simulink model "StepperMotorMusicPulseOutput4"  (R2019b)
settings: Solver=FixedStepDiscrete  StartTime=0.0  StopTime=t_sim  FixedStep=T_s  RelTol=1e-3  EnableMultiTasking=on
undefined symbols (not defined in the file): T_s, t_sim
libraries: dspsigops x10, sbox2 x3
settings Model: Creator=haketa  LastModifiedBy=STEPPERMOTOR
settings DataIOCC: LimitDataPoints=on  SaveFormat=Array  SignalLoggingSaveFormat=ModelDataLogs  ReturnWorkspaceOutputs=off
settings OptimizationCC: BlockReduction=off  OptimizeBlockIOStorage=off  BufferReuse=off  GlobalBufferReuse=off  ExpressionFolding=off  ExpressionDepthLimit=2147483647  LocalBlockOutputs=off  InitFltsAndDblsToZero=on  LifeSpan=inf  OptimizeDataStoreBuffers=off  BusAssignmentInplaceUpdate=off
settings DebuggingCC: SaveWithParameterizedLinksMsg=none  UnderspecifiedInitializationDetection=Classic  MergeDetectMultiDrivingBlocksExec=none  SignalResolutionControl=TryResolveAllWithWarning  SolverPrmCheckMsg=warning  InheritedTsInSrcMsg=none  MultiTaskDSMMsg=warning  MultiTaskCondExecSysMsg=none  FcnCallInpInsideContextMsg=warning  StateNameClashWarn=warning  SFUnexpectedBacktrackingDiag=warning  SFNoUnconditionalDefaultTransitionDiag=warning  SFExecutionAtInitializationDiag=none  ArithmeticOperatorsInVariantConditions=warning
settings HardwareCC: ProdBitPerPointer=32  ProdBitPerSizeT=32  ProdBitPerPtrDiffT=32  ProdLargestAtomicFloat=None  ProdIntDivRoundTo=Undefined  ProdEndianess=Unspecified  ProdWordSize=32  ProdHWDeviceType=32-bit Generic
settings ModelReferenceCC: PropagateSignalLabelsOutOfModel=off
settings SFSimCC: SimUseLocalCustomCode=off  CustomCodeUndefinedFunction=UseInterfaceOnly
settings RTWCC: Description=MTT sBOXII Real-Time Target.  SystemTargetFile=sbox2.tlc  TemplateMakefile=sbox2.tmf  RTWUseLocalCustomCode=off  RTWCompilerOptimization=on
settings CodeAppCC: StateflowObjectComments=on
settings GRTTargetCC: TargetLangStandard=C89/C90 (ANSI)  GeneratePreprocessorConditionals=Disable all  MatFileLogging=off  UseToolchainInfoCompliant=off  RTWCAPISignals=on  RTWCAPIParams=on
settings ConfigComp: CovMetricSettings=dw  CovHtmlReporting=on  CovSaveCumulativeToWorkspaceVar=on  CovSaveSingleToWorkspaceVar=on  CovExternalEMLEnable=off  CovSFcnEnable=off

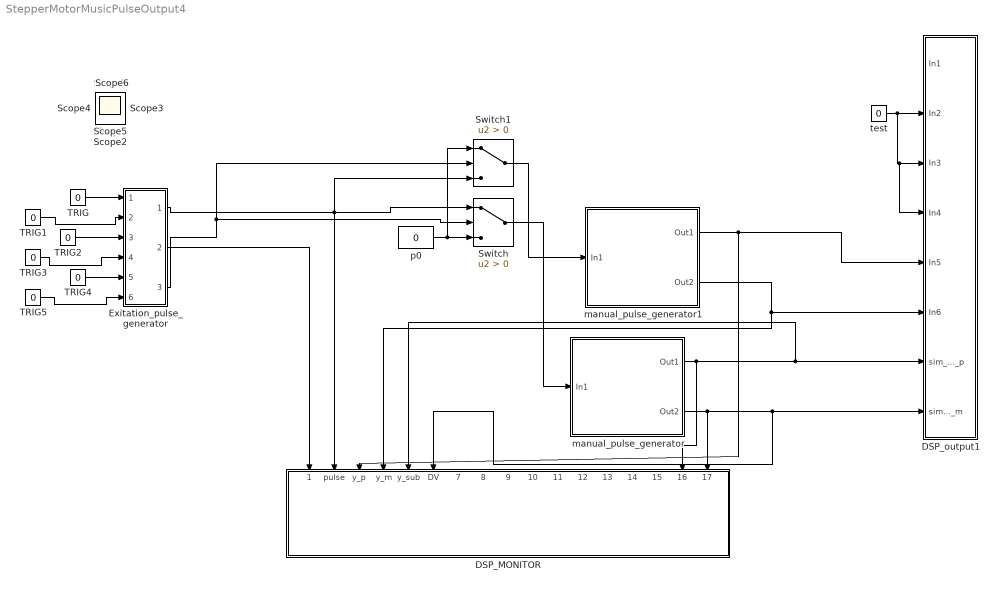
== system StepperMotorMusicPulseOutput4 ==
  DSP_MONITOR : Subsystem
  DSP_output1 : Subsystem
  Exitation_pulse_generator : Subsystem
  Switch : Switch  Criteria=u2 > Threshold
  Switch1 : Switch  Criteria=u2 > Threshold
  TRIG{,1..5} (6 alike) : Constant  Value=0  SampleTime=-1
  manual_pulse_generator : Subsystem
  manual_pulse_generator1 : Subsystem
  p0 : Constant  Value=0  SampleTime=-1
  test : Constant  Value=0  SampleTime=-1
  Scope{,1..6} (7 alike) : Scope
  wires:
  TRIG/1 -> Exitation_pulse_generator/1(TRIG)
  TRIG1/1 -> Exitation_pulse_generator/2(In2)
  TRIG3/1 -> Exitation_pulse_generator/4(In4)
  manual_pulse_generator/2(Out2) -> DSP_MONITOR/6(DV), DSP_output1/8(sim_CW_m), DSP_MONITOR/17(hoge2)
  manual_pulse_generator/1(Out1) -> DSP_output1/7(sim_CW_p), DSP_MONITOR/5(y_sub), DSP_MONITOR/16(hoge1)
  Exitation_pulse_generator/2(TRIG_parameter) -> DSP_MONITOR/1(DSP_SAVE_TRIG)
  Exitation_pulse_generator/1(sim_CW) -> Switch/1, Switch1/3, DSP_MONITOR/2(pulse)
  test/1 -> DSP_output1/2(In2), DSP_output1/3(In3), DSP_output1/4(In4)
  TRIG2/1 -> Exitation_pulse_generator/3(In3)
  TRIG4/1 -> Exitation_pulse_generator/5(In5)
  TRIG5/1 -> Exitation_pulse_generator/6(CW_p)
  Exitation_pulse_generator/3("Rot ") -> Switch/2, Switch1/2
  p0/1 -> Switch1/1, Switch/3
  Switch1/1 -> manual_pulse_generator1/1(In1)
  Switch/1 -> manual_pulse_generator/1(In1)
  manual_pulse_generator1/1(Out1) -> DSP_output1/5(In5), DSP_MONITOR/3(y_p)
  manual_pulse_generator1/2(Out2) -> DSP_MONITOR/4(y_m), DSP_output1/6(In6)

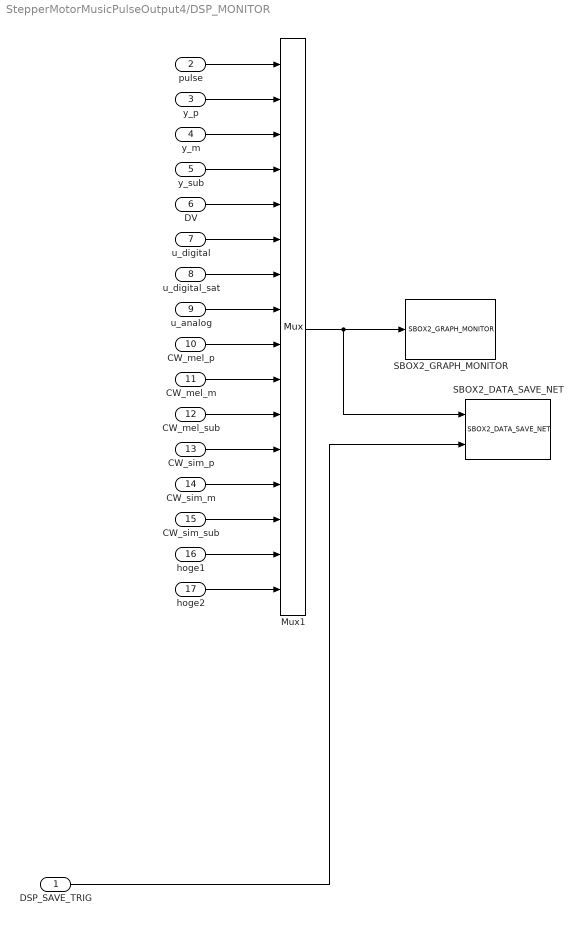
== system StepperMotorMusicPulseOutput4/DSP_MONITOR ==
  DSP_SAVE_TRIG : Inport
  pulse : Inport  Port=2
  y_p : Inport  Port=3
  y_m : Inport  Port=4
  y_sub : Inport  Port=5
  DV : Inport  Port=6
  u_digital : Inport  Port=7
  u_digital_sat : Inport  Port=8
  u_analog : Inport  Port=9
  CW_mel_p : Inport  Port=10
  CW_mel_m : Inport  Port=11
  CW_mel_sub : Inport  Port=12
  CW_sim_p : Inport  Port=13
  CW_sim_m : Inport  Port=14
  CW_sim_sub : Inport  Port=15
  hoge1 : Inport  Port=16
  hoge2 : Inport  Port=17
  Mux1 : Mux  Inputs=16
  SBOX2_DATA_SAVE_NET : sbox2/Network Data Save Devices/SBOX2_DATA_SAVE_NET  save_mode=ホストアプリケーション指示によるトリガ待ち  data_length=(t_sim/T_s)  pre_triger=0  sampletime=-1
  SBOX2_GRAPH_MONITOR : sbox2/Network Data Save Devices/SBOX2_GRAPH_MONITOR  sampletime=-1
  wires:
  DSP_SAVE_TRIG/1 -> SBOX2_DATA_SAVE_NET/2
  y_p/1 -> Mux1/2
  Mux1/1 -> SBOX2_DATA_SAVE_NET/1, SBOX2_GRAPH_MONITOR/1
  pulse/1 -> Mux1/1
  y_sub/1 -> Mux1/4
  u_digital/1 -> Mux1/6
  u_analog/1 -> Mux1/8
  u_digital_sat/1 -> Mux1/7
  DV/1 -> Mux1/5
  y_m/1 -> Mux1/3
  CW_mel_p/1 -> Mux1/9
  CW_mel_m/1 -> Mux1/10
  CW_mel_sub/1 -> Mux1/11
  CW_sim_p/1 -> Mux1/12
  CW_sim_m/1 -> Mux1/13
  CW_sim_sub/1 -> Mux1/14
  hoge1/1 -> Mux1/15
  hoge2/1 -> Mux1/16

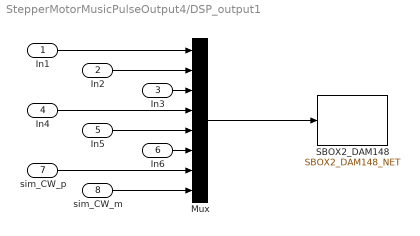
== system StepperMotorMusicPulseOutput4/DSP_output1 ==
  In1 : Inport
  In2 : Inport  Port=2
  In3 : Inport  Port=3
  In4 : Inport  Port=4
  In5 : Inport  Port=5
  In6 : Inport  Port=6
  sim_CW_p : Inport  Port=7
  sim_CW_m : Inport  Port=8
  Mux : Mux  Inputs=8
  SBOX2_DAM148 : sbox2/Analog I//O Devices/SBOX2_DAM148_NET  daStopCtrl1=0V出力  daStopCtrl2=0V出力  daStopCtrl3=0V出力  daStopCtrl4=0V出力  daStopCtrl5=0V出力  daStopCtrl6=0V出力  daStopCtrl7=0V出力  daStopCtrl8=0V出力  sampletime=-1
  wires:
  sim_CW_p/1 -> Mux/7
  Mux/1 -> SBOX2_DAM148/1
  In2/1 -> Mux/2
  In1/1 -> Mux/1
  In4/1 -> Mux/4
  In5/1 -> Mux/5
  In6/1 -> Mux/6
  sim_CW_m/1 -> Mux/8
  In3/1 -> Mux/3

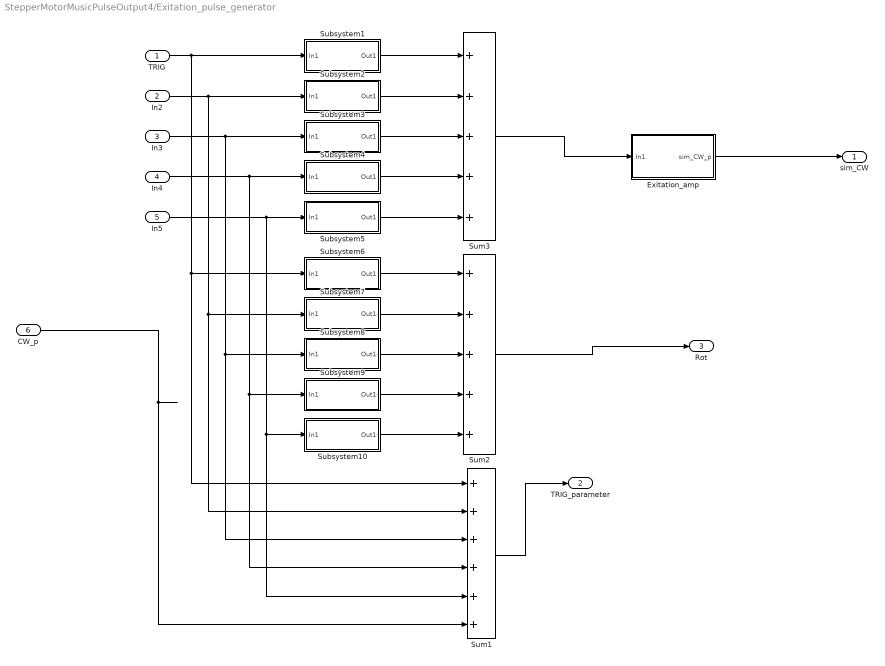
== system StepperMotorMusicPulseOutput4/Exitation_pulse_generator ==
  TRIG : Inport
  In2 : Inport  Port=2
  In3 : Inport  Port=3
  In4 : Inport  Port=4
  In5 : Inport  Port=5
  CW_p : Inport  Port=6
  Exitation_amp : Subsystem
  Subsystem1 : Subsystem
  Subsystem10 : Subsystem
  Subsystem2 : Subsystem
  Subsystem3 : Subsystem
  Subsystem4 : Subsystem
  Subsystem5 : Subsystem
  Subsystem6 : Subsystem
  Subsystem7 : Subsystem
  Subsystem8 : Subsystem
  Subsystem9 : Subsystem
  Sum1 : Sum  Inputs=++++++
  Sum2 : Sum  Inputs=+++++
  Sum3 : Sum  Inputs=+++++
  sim_CW : Outport
  TRIG_parameter : Outport  Port=2
  "Rot " : Outport  Port=3
  wires:
  Sum3/1 -> Exitation_amp/1(In1)
  Exitation_amp/1(sim_CW_p) -> sim_CW/1
  Subsystem1/1(Out1) -> Sum3/1
  In2/1 -> Subsystem2/1(In1), Sum1/2, Subsystem7/1(In1)
  In3/1 -> Subsystem3/1(In1), Subsystem8/1(In1), Sum1/3
  In4/1 -> Subsystem4/1(In1), Sum1/4, Subsystem9/1(In1)
  In5/1 -> Subsystem5/1(In1), Subsystem10/1(In1), Sum1/5
  CW_p/1 -> Sum1/6
  Subsystem2/1(Out1) -> Sum3/2
  Subsystem3/1(Out1) -> Sum3/3
  Subsystem4/1(Out1) -> Sum3/4
  Subsystem5/1(Out1) -> Sum3/5
  TRIG/1 -> Subsystem1/1(In1), Sum1/1, Subsystem6/1(In1)
  Subsystem7/1(Out1) -> Sum2/2
  Subsystem8/1(Out1) -> Sum2/3
  Subsystem9/1(Out1) -> Sum2/4
  Sum1/1 -> TRIG_parameter/1
  Subsystem10/1(Out1) -> Sum2/5
  Subsystem6/1(Out1) -> Sum2/1
  Sum2/1 -> "Rot "/1

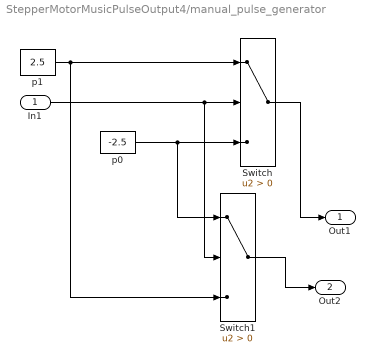
== system StepperMotorMusicPulseOutput4/manual_pulse_generator ==
  In1 : Inport
  Switch : Switch  Criteria=u2 > Threshold
  Switch1 : Switch  Criteria=u2 > Threshold
  p0 : Constant  Value=-2.5  SampleTime=-1
  p1 : Constant  Value=2.5  SampleTime=-1
  Out1 : Outport
  Out2 : Outport  Port=2
  wires:
  Switch1/1 -> Out2/1
  In1/1 -> Switch1/2, Switch/2
  Switch/1 -> Out1/1
  p1/1 -> Switch1/3, Switch/1
  p0/1 -> Switch1/1, Switch/3

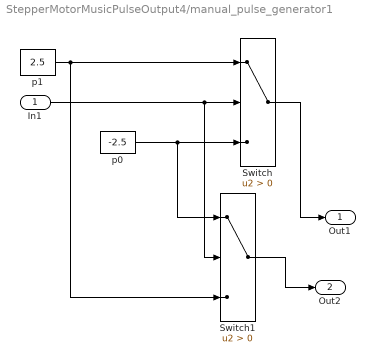
== system StepperMotorMusicPulseOutput4/manual_pulse_generator1 ==
  In1 : Inport
  Switch : Switch  Criteria=u2 > Threshold
  Switch1 : Switch  Criteria=u2 > Threshold
  p0 : Constant  Value=-2.5  SampleTime=-1
  p1 : Constant  Value=2.5  SampleTime=-1
  Out1 : Outport
  Out2 : Outport  Port=2
  wires:
  p0/1 -> Switch/3, Switch1/1
  p1/1 -> Switch/1, Switch1/3
  Switch/1 -> Out1/1
  In1/1 -> Switch/2, Switch1/2
  Switch1/1 -> Out2/1

== system StepperMotorMusicPulseOutput4/Exitation_pulse_generator/Exitation_amp ==
  In1 : Inport
  Constant3 : Constant  Value=4.5  SampleTime=-1
  Gain5 : Gain  Gain=-1
  Switch : Switch  Criteria=u2 > Threshold
  sim_CW_p : Outport
  wires:
  Constant3/1 -> Switch/1, Gain5/1
  Gain5/1 -> Switch/3  "DV"
  Switch/1 -> sim_CW_p/1
  In1/1 -> Switch/2

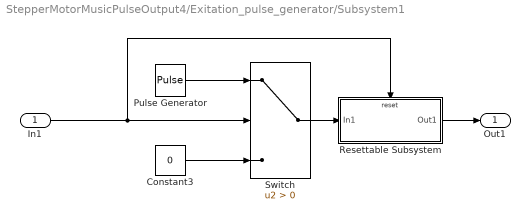
== system StepperMotorMusicPulseOutput4/Exitation_pulse_generator/Subsystem1 ==
  In1 : Inport
  Constant3 : Constant  Value=0  SampleTime=-1
  Pulse Generator : DiscretePulseGenerator  PulseType=Time based  Period=T_s*2  PulseWidth=50
  Resettable Subsystem : Subsystem  TreatAsAtomicUnit=on
  Switch : Switch  Criteria=u2 > Threshold
  Out1 : Outport
  wires:
  In1/1 -> Switch/2, Resettable Subsystem/Reset
  Pulse Generator/1 -> Switch/1
  Constant3/1 -> Switch/3
  Resettable Subsystem/1(Out1) -> Out1/1
  Switch/1 -> Resettable Subsystem/1(In1)

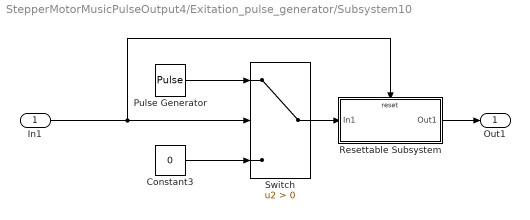
== system StepperMotorMusicPulseOutput4/Exitation_pulse_generator/Subsystem10 ==
  In1 : Inport
  Constant3 : Constant  Value=0  SampleTime=-1
  Pulse Generator : DiscretePulseGenerator  PulseType=Time based  Period=T_s*2  PulseWidth=50
  Resettable Subsystem : Subsystem  TreatAsAtomicUnit=on
  Switch : Switch  Criteria=u2 > Threshold
  Out1 : Outport
  wires:
  Switch/1 -> Resettable Subsystem/1(In1)
  Resettable Subsystem/1(Out1) -> Out1/1
  Constant3/1 -> Switch/3
  Pulse Generator/1 -> Switch/1
  In1/1 -> Resettable Subsystem/Reset, Switch/2

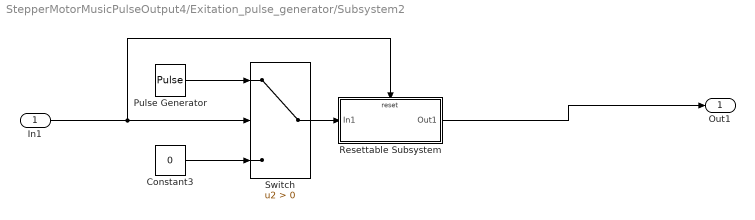
== system StepperMotorMusicPulseOutput4/Exitation_pulse_generator/Subsystem2 ==
  In1 : Inport
  Constant3 : Constant  Value=0  SampleTime=-1
  Pulse Generator : DiscretePulseGenerator  PulseType=Time based  Period=T_s*2  PulseWidth=50
  Resettable Subsystem : Subsystem  TreatAsAtomicUnit=on
  Switch : Switch  Criteria=u2 > Threshold
  Out1 : Outport
  wires:
  Switch/1 -> Resettable Subsystem/1(In1)
  Resettable Subsystem/1(Out1) -> Out1/1
  Constant3/1 -> Switch/3
  Pulse Generator/1 -> Switch/1
  In1/1 -> Resettable Subsystem/Reset, Switch/2

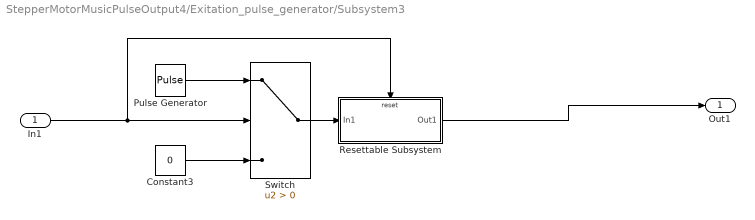
== system StepperMotorMusicPulseOutput4/Exitation_pulse_generator/Subsystem3 ==
  In1 : Inport
  Constant3 : Constant  Value=0  SampleTime=-1
  Pulse Generator : DiscretePulseGenerator  PulseType=Time based  Period=T_s*2  PulseWidth=50
  Resettable Subsystem : Subsystem  TreatAsAtomicUnit=on
  Switch : Switch  Criteria=u2 > Threshold
  Out1 : Outport
  wires:
  In1/1 -> Switch/2, Resettable Subsystem/Reset
  Pulse Generator/1 -> Switch/1
  Constant3/1 -> Switch/3
  Resettable Subsystem/1(Out1) -> Out1/1
  Switch/1 -> Resettable Subsystem/1(In1)

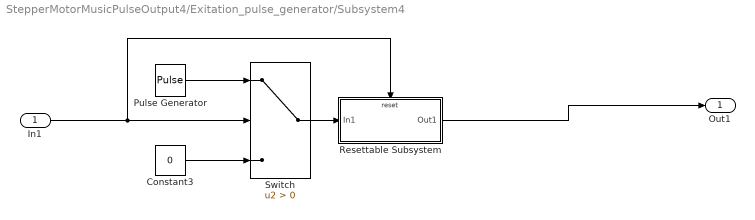
== system StepperMotorMusicPulseOutput4/Exitation_pulse_generator/Subsystem4 ==
  In1 : Inport
  Constant3 : Constant  Value=0  SampleTime=-1
  Pulse Generator : DiscretePulseGenerator  PulseType=Time based  Period=T_s*2  PulseWidth=50
  Resettable Subsystem : Subsystem  TreatAsAtomicUnit=on
  Switch : Switch  Criteria=u2 > Threshold
  Out1 : Outport
  wires:
  Switch/1 -> Resettable Subsystem/1(In1)
  Resettable Subsystem/1(Out1) -> Out1/1
  Constant3/1 -> Switch/3
  Pulse Generator/1 -> Switch/1
  In1/1 -> Resettable Subsystem/Reset, Switch/2

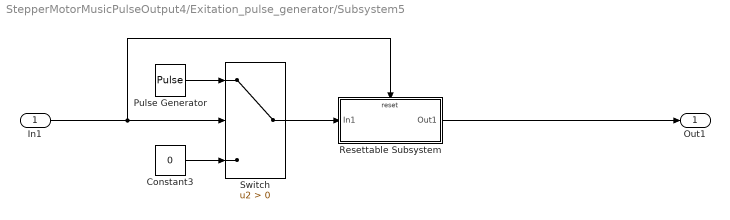
== system StepperMotorMusicPulseOutput4/Exitation_pulse_generator/Subsystem5 ==
  In1 : Inport
  Constant3 : Constant  Value=0  SampleTime=-1
  Pulse Generator : DiscretePulseGenerator  PulseType=Time based  Period=T_s*2  PulseWidth=50
  Resettable Subsystem : Subsystem  TreatAsAtomicUnit=on
  Switch : Switch  Criteria=u2 > Threshold
  Out1 : Outport
  wires:
  In1/1 -> Switch/2, Resettable Subsystem/Reset
  Pulse Generator/1 -> Switch/1
  Constant3/1 -> Switch/3
  Resettable Subsystem/1(Out1) -> Out1/1
  Switch/1 -> Resettable Subsystem/1(In1)

== system StepperMotorMusicPulseOutput4/Exitation_pulse_generator/Subsystem6 ==
  In1 : Inport
  Constant3 : Constant  Value=0  SampleTime=-1
  Pulse Generator : DiscretePulseGenerator  PulseType=Time based  Period=T_s*2  PulseWidth=50
  Resettable Subsystem : Subsystem  TreatAsAtomicUnit=on
  Switch : Switch  Criteria=u2 > Threshold
  Out1 : Outport
  wires:
  Switch/1 -> Resettable Subsystem/1(In1)
  Resettable Subsystem/1(Out1) -> Out1/1
  Constant3/1 -> Switch/3
  Pulse Generator/1 -> Switch/1
  In1/1 -> Resettable Subsystem/Reset, Switch/2

== system StepperMotorMusicPulseOutput4/Exitation_pulse_generator/Subsystem7 ==
  In1 : Inport
  Constant3 : Constant  Value=0  SampleTime=-1
  Pulse Generator : DiscretePulseGenerator  PulseType=Time based  Period=T_s*2  PulseWidth=50
  Resettable Subsystem : Subsystem  TreatAsAtomicUnit=on
  Switch : Switch  Criteria=u2 > Threshold
  Out1 : Outport
  wires:
  In1/1 -> Switch/2, Resettable Subsystem/Reset
  Pulse Generator/1 -> Switch/1
  Constant3/1 -> Switch/3
  Resettable Subsystem/1(Out1) -> Out1/1
  Switch/1 -> Resettable Subsystem/1(In1)

== system StepperMotorMusicPulseOutput4/Exitation_pulse_generator/Subsystem8 ==
  In1 : Inport
  Constant3 : Constant  Value=0  SampleTime=-1
  Pulse Generator : DiscretePulseGenerator  PulseType=Time based  Period=T_s*2  PulseWidth=50
  Resettable Subsystem : Subsystem  TreatAsAtomicUnit=on
  Switch : Switch  Criteria=u2 > Threshold
  Out1 : Outport
  wires:
  Switch/1 -> Resettable Subsystem/1(In1)
  Resettable Subsystem/1(Out1) -> Out1/1
  Constant3/1 -> Switch/3
  Pulse Generator/1 -> Switch/1
  In1/1 -> Resettable Subsystem/Reset, Switch/2

== system StepperMotorMusicPulseOutput4/Exitation_pulse_generator/Subsystem9 ==
  In1 : Inport
  Constant3 : Constant  Value=0  SampleTime=-1
  Pulse Generator : DiscretePulseGenerator  PulseType=Time based  Period=T_s*2  PulseWidth=50
  Resettable Subsystem : Subsystem  TreatAsAtomicUnit=on
  Switch : Switch  Criteria=u2 > Threshold
  Out1 : Outport
  wires:
  In1/1 -> Switch/2, Resettable Subsystem/Reset
  Pulse Generator/1 -> Switch/1
  Constant3/1 -> Switch/3
  Resettable Subsystem/1(Out1) -> Out1/1
  Switch/1 -> Resettable Subsystem/1(In1)

== system StepperMotorMusicPulseOutput4/Exitation_pulse_generator/Subsystem1/Resettable Subsystem ==
  In1 : Inport
  Reset : ResetPort  DisableCoverage=on  ResetTriggerType=falling
  Triggered Signal From Workspace : dspsigops/Triggered Signal From Workspace  Signal=MusicPulse  TriggerType=Either edge  ic=0  SamplesPerFrame=1  OutputAfterFinalValue=Setting to zero  OutputFrames=off
      settings: SourceProductName=DSP System Toolbox  SourceProductBaseCode=DS
  Out1 : Outport
  wires:
  In1/1 -> Triggered Signal From Workspace/Trigger
  Triggered Signal From Workspace/1 -> Out1/1

== system StepperMotorMusicPulseOutput4/Exitation_pulse_generator/Subsystem10/Resettable Subsystem ==
  In1 : Inport
  Reset : ResetPort  DisableCoverage=on  ResetTriggerType=falling
  Triggered Signal From Workspace : dspsigops/Triggered Signal From Workspace  Signal=DoR  TriggerType=Either edge  ic=0  SamplesPerFrame=1  OutputAfterFinalValue=Setting to zero  OutputFrames=off
      settings: SourceProductName=DSP System Toolbox  SourceProductBaseCode=DS
  Out1 : Outport
  wires:
  Triggered Signal From Workspace/1 -> Out1/1
  In1/1 -> Triggered Signal From Workspace/Trigger

== system StepperMotorMusicPulseOutput4/Exitation_pulse_generator/Subsystem2/Resettable Subsystem ==
  In1 : Inport
  Reset : ResetPort  DisableCoverage=on  ResetTriggerType=falling
  Triggered Signal From Workspace : dspsigops/Triggered Signal From Workspace  Signal=MusicPulse  TriggerType=Either edge  ic=0  SamplesPerFrame=1  OutputAfterFinalValue=Setting to zero  OutputFrames=off
      settings: SourceProductName=DSP System Toolbox  SourceProductBaseCode=DS
  Out1 : Outport
  wires:
  Triggered Signal From Workspace/1 -> Out1/1
  In1/1 -> Triggered Signal From Workspace/Trigger

== system StepperMotorMusicPulseOutput4/Exitation_pulse_generator/Subsystem3/Resettable Subsystem ==
  In1 : Inport
  Reset : ResetPort  DisableCoverage=on  ResetTriggerType=falling
  Triggered Signal From Workspace : dspsigops/Triggered Signal From Workspace  Signal=MusicPulse  TriggerType=Either edge  ic=0  SamplesPerFrame=1  OutputAfterFinalValue=Setting to zero  OutputFrames=off
      settings: SourceProductName=DSP System Toolbox  SourceProductBaseCode=DS
  Out1 : Outport
  wires:
  In1/1 -> Triggered Signal From Workspace/Trigger
  Triggered Signal From Workspace/1 -> Out1/1

== system StepperMotorMusicPulseOutput4/Exitation_pulse_generator/Subsystem4/Resettable Subsystem ==
  In1 : Inport
  Reset : ResetPort  DisableCoverage=on  ResetTriggerType=falling
  Triggered Signal From Workspace : dspsigops/Triggered Signal From Workspace  Signal=MusicPulse  TriggerType=Either edge  ic=0  SamplesPerFrame=1  OutputAfterFinalValue=Setting to zero  OutputFrames=off
      settings: SourceProductName=DSP System Toolbox  SourceProductBaseCode=DS
  Out1 : Outport
  wires:
  Triggered Signal From Workspace/1 -> Out1/1
  In1/1 -> Triggered Signal From Workspace/Trigger

== system StepperMotorMusicPulseOutput4/Exitation_pulse_generator/Subsystem5/Resettable Subsystem ==
  In1 : Inport
  Reset : ResetPort  DisableCoverage=on  ResetTriggerType=falling
  Triggered Signal From Workspace : dspsigops/Triggered Signal From Workspace  Signal=MusicPulse  TriggerType=Either edge  ic=0  SamplesPerFrame=1  OutputAfterFinalValue=Setting to zero  OutputFrames=off
      settings: SourceProductName=DSP System Toolbox  SourceProductBaseCode=DS
  Out1 : Outport
  wires:
  In1/1 -> Triggered Signal From Workspace/Trigger
  Triggered Signal From Workspace/1 -> Out1/1

== system StepperMotorMusicPulseOutput4/Exitation_pulse_generator/Subsystem6/Resettable Subsystem ==
  In1 : Inport
  Reset : ResetPort  DisableCoverage=on  ResetTriggerType=falling
  Triggered Signal From Workspace : dspsigops/Triggered Signal From Workspace  Signal=DoR  TriggerType=Either edge  ic=0  SamplesPerFrame=1  OutputAfterFinalValue=Setting to zero  OutputFrames=off
      settings: SourceProductName=DSP System Toolbox  SourceProductBaseCode=DS
  Out1 : Outport
  wires:
  Triggered Signal From Workspace/1 -> Out1/1
  In1/1 -> Triggered Signal From Workspace/Trigger

== system StepperMotorMusicPulseOutput4/Exitation_pulse_generator/Subsystem7/Resettable Subsystem ==
  In1 : Inport
  Reset : ResetPort  DisableCoverage=on  ResetTriggerType=falling
  Triggered Signal From Workspace : dspsigops/Triggered Signal From Workspace  Signal=DoR  TriggerType=Either edge  ic=0  SamplesPerFrame=1  OutputAfterFinalValue=Setting to zero  OutputFrames=off
      settings: SourceProductName=DSP System Toolbox  SourceProductBaseCode=DS
  Out1 : Outport
  wires:
  In1/1 -> Triggered Signal From Workspace/Trigger
  Triggered Signal From Workspace/1 -> Out1/1

== system StepperMotorMusicPulseOutput4/Exitation_pulse_generator/Subsystem8/Resettable Subsystem ==
  In1 : Inport
  Reset : ResetPort  DisableCoverage=on  ResetTriggerType=falling
  Triggered Signal From Workspace : dspsigops/Triggered Signal From Workspace  Signal=DoR  TriggerType=Either edge  ic=0  SamplesPerFrame=1  OutputAfterFinalValue=Setting to zero  OutputFrames=off
      settings: SourceProductName=DSP System Toolbox  SourceProductBaseCode=DS
  Out1 : Outport
  wires:
  Triggered Signal From Workspace/1 -> Out1/1
  In1/1 -> Triggered Signal From Workspace/Trigger

== system StepperMotorMusicPulseOutput4/Exitation_pulse_generator/Subsystem9/Resettable Subsystem ==
  In1 : Inport
  Reset : ResetPort  DisableCoverage=on  ResetTriggerType=falling
  Triggered Signal From Workspace : dspsigops/Triggered Signal From Workspace  Signal=DoR  TriggerType=Either edge  ic=0  SamplesPerFrame=1  OutputAfterFinalValue=Setting to zero  OutputFrames=off
      settings: SourceProductName=DSP System Toolbox  SourceProductBaseCode=DS
  Out1 : Outport
  wires:
  In1/1 -> Triggered Signal From Workspace/Trigger
  Triggered Signal From Workspace/1 -> Out1/1
